simulink model "verify_Pipe_Biflow_mdl"  (R2018b)
settings: Solver=VariableStepAuto  StartTime=0.0  StopTime=24*3600  MaxStep=100  RelTol=1e-3  EnableMultiTasking=on
undefined symbols (not defined in the file or in its folder): path_carnot
libraries: carnot x5, simulink x2
settings Model: Creator=drhf  LastModifiedBy=P41573
settings DataIOCC: SaveFormat=Array  SignalLoggingSaveFormat=ModelDataLogs
settings OptimizationCC: ExpressionDepthLimit=2147483647  LifeSpan=inf
settings DebuggingCC: UnderspecifiedInitializationDetection=Classic  MergeDetectMultiDrivingBlocksExec=none  SolverPrmCheckMsg=warning  FcnCallInpInsideContextMsg=warning  StateNameClashWarn=warning  SFUnexpectedBacktrackingDiag=warning  SFNoUnconditionalDefaultTransitionDiag=warning  SFExecutionAtInitializationDiag=none
settings HardwareCC: ProdBitPerPointer=32  ProdBitPerSizeT=32  ProdBitPerPtrDiffT=32  ProdLargestAtomicFloat=None  ProdIntDivRoundTo=Undefined  ProdEndianess=Unspecified  ProdWordSize=32  ProdHWDeviceType=32-bit Generic
settings ModelReferenceCC: PropagateSignalLabelsOutOfModel=off
settings SFSimCC: SimUseLocalCustomCode=off
settings RTWCC: RTWUseLocalCustomCode=off
settings CodeAppCC: StateflowObjectComments=on
settings GRTTargetCC: TargetLangStandard=C89/C90 (ANSI)  GeneratePreprocessorConditionals=Disable all  CombineOutputUpdateFcns=off  GRTInterface=on
settings ConfigComp: CovMetricSettings=dw  CovHtmlReporting=on  CovSaveCumulativeToWorkspaceVar=on  CovSaveSingleToWorkspaceVar=on  CovExternalEMLEnable=off

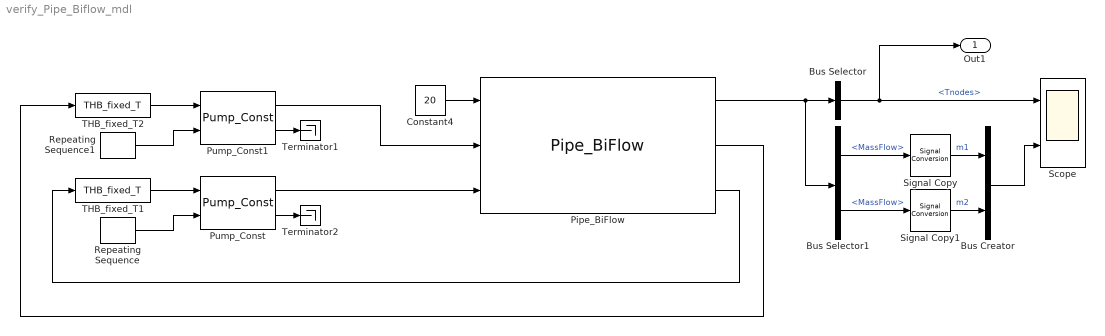
== system verify_Pipe_Biflow_mdl ==
  Bus Creator : BusCreator  Inputs=2
  Bus Selector : BusSelector  OutputSignals=Tnodes
  Bus Selector1 : BusSelector  OutputSignals=THBout_pipe1.MassFlow,THBin_pipe2.MassFlow
  Constant4 : Constant  Value=20
  Pipe_BiFlow : carnot/Hydraulics/Pipe_BiFlow  t0=20  hgt=318.3099  tini=[20 20 20 20 20 20 20 20 20 20 20 20 20 20 20 20 20 20 20 20 20 20 20 20 20 20 20 20 20 20 20 20 20 20 20 20 20 20 20 20 20 20 20 20 20 20 20 20 20 20 20 20 20 20 20 20 20 20 20 20 20 20 20 20 20 20 20 20 20 20 20 20 20 20 20 20 20 20 20 20 20 20 20 20 20 20 20 20 20 20 20 20 20 20 20 20 20 20 20 20]  mpts=[5 15 25 35 45 55 65 75 85 95]  PathName=fullfile(path_carnot('libsl'),'Hydraulics','Pipe_BiFlow','parameter_set')  FileName='PipeBF_NoLoss.mat'  userPath=off  userParam=off  uwall=0  ubot=0  utop=0  axcond=0  volume=10  dia=0.2  standing=standing cylinder  nodes=100  mpoints=10  pipe1inlet=1  pipe1outlet=0  pipe1dia=0.1  pipe2inlet=0  pipe2outlet=1  pipe2dia=0.1
      settings: SourceProductName=Carnot
  Pump_Const : carnot/Hydraulics/Pump_Const  mdotmax=0.5  dia=0.02  p0=3e5  fluid_id=Water  mix=0  mix2=0  mix3=0  UA=3  mcp=4182  Tini=20  e0=10  e1=10  e2=-1
      settings: SourceProductName=Carnot
  Pump_Const1 : carnot/Hydraulics/Pump_Const  mdotmax=0.4  dia=0.02  p0=3e5  fluid_id=Water  mix=0  mix2=0  mix3=0  UA=3  mcp=4182  Tini=20  e0=10  e1=10  e2=-1
      settings: SourceProductName=Carnot
  Repeating Sequence : simulink/Sources/Repeating Sequence  rep_seq_t=[0 10.5 11.5 24]*3600  rep_seq_y=[1 1 0 0]
  Repeating Sequence1 : simulink/Sources/Repeating Sequence  rep_seq_t=[0 10.5 11.5 24]*3600  rep_seq_y=[0 0 1 1]
  Scope : Scope  NumInputPorts=2
  Signal Copy : SignalConversion  OverrideOpt=off
  Signal Copy1 : SignalConversion  OverrideOpt=off
  THB_fixed_T1 : carnot/Source/Simple/THB_fixed_T  t=60
      settings: SourceProductName=Carnot
  THB_fixed_T2 : carnot/Source/Simple/THB_fixed_T  t=40
      settings: SourceProductName=Carnot
  Terminator1 : Terminator
  Terminator2 : Terminator
  Out1 : Outport
  wires:
  Pipe_BiFlow/3 -> THB_fixed_T1/1
  Pump_Const/2 -> Terminator2/1
  Pump_Const1/2 -> Terminator1/1
  Bus Creator/1 -> Scope/2
  Signal Copy/1 -> Bus Creator/1  "m1"
  Bus Selector1/2 -> Signal Copy1/1  "<MassFlow>"
  Bus Selector1/1 -> Signal Copy/1  "<MassFlow>"
  Pump_Const1/1 -> Pipe_BiFlow/2
  Bus Selector/1 -> Out1/1, Scope/1  "<Tnodes>"
  Signal Copy1/1 -> Bus Creator/2  "m2"
  THB_fixed_T1/1 -> Pump_Const/1
  Pump_Const/1 -> Pipe_BiFlow/3
  Repeating Sequence/1 -> Pump_Const/2
  Repeating Sequence1/1 -> Pump_Const1/2
  THB_fixed_T2/1 -> Pump_Const1/1
  Pipe_BiFlow/2 -> THB_fixed_T2/1
  Constant4/1 -> Pipe_BiFlow/1
  Pipe_BiFlow/1 -> Bus Selector1/1, Bus Selector/1
